simulink model "Problem5"  (R2021a)
settings: Solver=VariableStepAuto  StartTime=0.0  StopTime=10.0  RelTol=1e-3
settings Model: Creator=Nida  LastModifiedBy=Nida

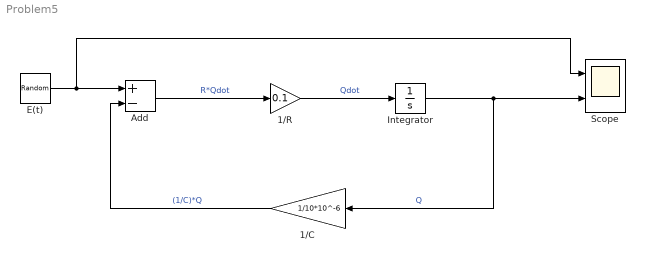
== system Problem5 ==
  1/C : Gain  Gain=1/10*10^-6
  1/R : Gain  Gain=0.1
  Add : Sum  Inputs=+-
  E(t) : RandomNumber  SampleTime=0.1
  Integrator : Integrator
  Scope : Scope  NumInputPorts=2
  wires:
  1/C/1 -> Add/2  "(1/C)*Q"
  Integrator/1 -> Scope/2, 1/C/1  "Q"
  E(t)/1 -> Scope/1, Add/1
  Add/1 -> 1/R/1  "R*Qdot"
  1/R/1 -> Integrator/1  "Qdot"
